simulink model "psbswitching"  (Simulink 6.0)
settings: Solver=ode15s  SolverMode=SingleTasking  StartTime=0.0  StopTime=.2  RelTol=1e-4
libraries: powerlib2 x12, powerlib_extras x1
settings Model: Creator=patrice  LastModifiedBy=batserve  ExtModeTrigMode=oneshot  ExtModeArmWhenConnect=off  ExtModeAutoUpdateStatusClock=off
settings DataIOCC: LimitDataPoints=off  SignalLoggingName=sigsOut
settings OptimizationCC: BlockReduction=off  BooleanDataType=off
settings DebuggingCC: CheckExecutionContextPreStartOutputMsg=on  CheckExecutionContextRuntimeOutputMsg=on  SolverPrmCheckMsg=none  UnconnectedInputMsg=none  UnconnectedOutputMsg=none
settings HardwareCC: TargetUnknown=on
settings RTWCC: TemplateMakefile=grt_vc.tmf

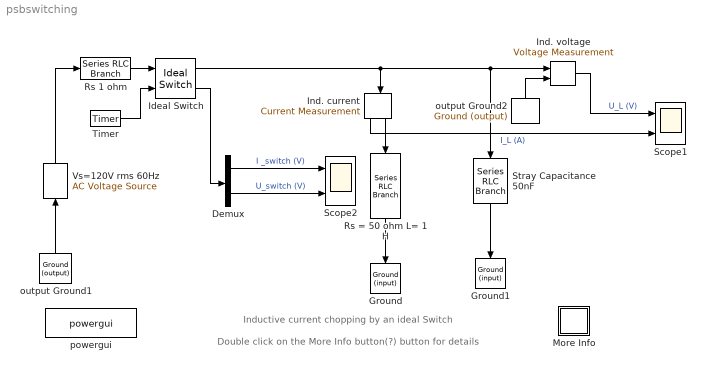
== system psbswitching ==
  note: Inductive current chopping by an ideal Switch
  note: Double click on the More Info button(?) button for details
  "  Ind. current" : powerlib2/Measurements/Current Measurement  Tag=PoWeRsYsTeMmEaSuReMeNt  Orientation=down  PhasorSimulation=off  OutputType=Magnitude  PSBOutputType=01  PSBequivalent=0
  Demux : Demux  Outputs=2
  Ground : powerlib2/Connectors/Ground (input)  Tag=PoWeRsYsTeMbLoCk  Orientation=down
  Ground1 : powerlib2/Connectors/Ground (input)  Tag=PoWeRsYsTeMbLoCk  Orientation=down
  Ideal Switch : powerlib2/Power Electronics/Ideal Switch  Tag=PoWeRsYsTeMbLoCk  Ron=1e-3  Lon=1e-9  IC=1  Rs=Inf  Cs=0  PSBOutputType=10
  Ind. voltage : powerlib2/Measurements/Voltage Measurement  Tag=PoWeRsYsTeMmEaSuReMeNt  PhasorSimulation=off  OutputType=Magnitude  PSBOutputType=0  PSBequivalent=0
  More Info : Subsystem
      mask Display: disp('?')
  Rs 1 ohm : powerlib2/Elements/Series RLC Branch  Tag=PoWeRsYsTeMbLoCk  a=1  b=0  c=Inf  mesure=None  PSBOutputType=1
  Rs = 50 ohm L= 1 H : powerlib2/Elements/Series RLC Branch  Tag=PoWeRsYsTeMbLoCk  Orientation=down  a=50  b=1  c=Inf  mesure=None  PSBOutputType=1
  Scope1 : Scope  NumInputPorts=2
      settings: TimeRange=0.2  YMin=-1000~-0.477505  YMax=1000~0.928922  SaveName=U_L  DataFormat=Array
  Scope2 : Scope  NumInputPorts=2
      settings: TimeRange=0.2  YMin=-30~-1000  YMax=10~1000  DataFormat=Array
  Stray Capacitance 50nF : powerlib2/Elements/Series RLC Branch  Tag=PoWeRsYsTeMbLoCk  Orientation=down  a=0  b=0  c=50e-9  mesure=None  PSBOutputType=1
  Timer : powerlib_extras/Control  Blocks/Timer  t=[0 36e-3 150e-3]  e=[1 0 1 ]
  Vs=120V rms 60Hz : powerlib2/Electrical Sources/AC Voltage Source  Tag=PoWeRsYsTeMbLoCk  Orientation=up  A=120*sqrt(2)  P=0  F=60  stime=0  mesure=None  PSBOutputType=1
  output Ground1 : powerlib2/Connectors/Ground (output)  Tag=PoWeRsYsTeMbLoCk  Orientation=up  PSBOutputType=1
  output Ground2 : powerlib2/Connectors/Ground (output)  Tag=PoWeRsYsTeMbLoCk  Orientation=up  PSBOutputType=1
  powergui : powerlib2/powergui  Frange=logspace(0,3,50)  Ylog=off  Xlog=off  save=off  variable=ZData  ZoomFFT=on  StartTime=0.0  cycles=1  DisplayStyle=off  fundamental=60  FreqAxis=off  MaxFrequency=1000  frequencyindice=1  frequencyindicesteady=1  RmsSteady=1  display=off  Ts=0  methode=off  frequency=60  echomessages=off
  wires:
  Ind. voltage/1 -> Scope1/1  "U_L (V)"
  Rs 1 ohm/1 -> Ideal Switch/1
  Timer/1 -> Ideal Switch/2
  Vs=120V rms 60Hz/1 -> Rs 1 ohm/1
  output Ground1/1 -> Vs=120V rms 60Hz/1
  "  Ind. current"/2 -> Rs = 50 ohm L= 1 H/1
  Stray Capacitance 50nF/1 -> Ground1/1
  output Ground2/1 -> Ind. voltage/2
  Ideal Switch/2 -> Demux/1
  Rs = 50 ohm L= 1 H/1 -> Ground/1
  "  Ind. current"/1 -> Scope1/2  "I_L (A)"
  Demux/1 -> Scope2/1  "I _switch (V)"
  Demux/2 -> Scope2/2  "U_switch (V)"
  Ideal Switch/1 -> "  Ind. current"/1, Ind. voltage/1, Stray Capacitance 50nF/1

== system psbswitching/More Info ==
  note: This example illustrates the effect of current chopping in an inductive circuit
  note: Circuit Description
  note: The  Ideal Switch is used to switch off and on an  inductor (L = 1H, R = 50 ohms) on a 120 Vrms,  60 Hz source.
      | The inductor has a stray capacitance C = 50 nF. The switch resistance  is 1e-3 ohm.
      | The switch is initially closed (initial state = 1). It is open at time t = 36ms and then reclosed at time t = 0.15 s.
  note: Demonstration
  note: G. Sybille (Hydro-Quebec)
  note: Start the simulation.and observe the inductor voltage U_L and inductor  current I_L  on Scope1
      | At the opening time, t = 36 ms, the current in the inductor is I_L= 0.187 A. The current chopping  in the inductor produces a
      | high  frequency overvoltage (711 Hz) across the inductor. The maximum voltage can be calculated from the following equation:
      |
      |      U_Lmax = I_L*sqrt(L/C) = 0.187*sqrt(1/50e-9) =  836 V
      |
      | At the reclosing time, t = 0.15 s , the source voltage is zero. Therefore, a full offset is observed in the inductor current.
      | The switch current spike observed on trace 1 of Scope2 at switch reclosing (t = 0.15 s) is due to the capacitor discharge through
      | the source resistance. If you zoom on this current spike you will observe a current step of 30 A
      | (30V capacitor voltage / 1 ohm source resistance), followed by a fast discharge time constant (RC = 1*50e-9 = 50e-9 s).
